simulink model "dspsdadc_fixpt"  (Simulink 8.3)
settings: Solver=ode5  SolverMode=SingleTasking  StartTime=0.0  StopTime=inf  MaxStep=1/512000  RelTol=1e-3  AbsTol=1e-6
libraries: dsparch4 x1, dspmlti4 x1, dspmisc x1
settings Model: Creator=The MathWorks Inc.  ExtModeTrigMode=oneshot  ExtModeArmWhenConnect=off  ExtModeAutoUpdateStatusClock=off
settings DataIOCC: LimitDataPoints=off  SignalLoggingSaveFormat=Dataset  SaveOutput=off  SaveTime=off  SignalLoggingName=logsOut
settings OptimizationCC: BlockReduction=off  BooleanDataType=off  ExpressionDepthLimit=2147483647  RollThreshold=2  InitFltsAndDblsToZero=on  EfficientMapNaN2IntZero=off
settings DebuggingCC: SaveWithParameterizedLinksMsg=none  SignalResolutionControl=TryResolveAllWithWarning  SolverPrmCheckMsg=none  MultiTaskDSMMsg=warning  MultiTaskCondExecSysMsg=none  IntegerOverflowMsg=none  ParameterPrecisionLossMsg=none  FcnCallInpInsideContextMsg=UseLocalSettings  StrictBusMsg=None  LoggingUnavailableSignals=none
settings HardwareCC: TargetUnknown=on
settings RTWCC: IncludeERTFirstTime=on
settings GRTTargetCC: TargetFcnLib=ansi_tfl_tmw.mat

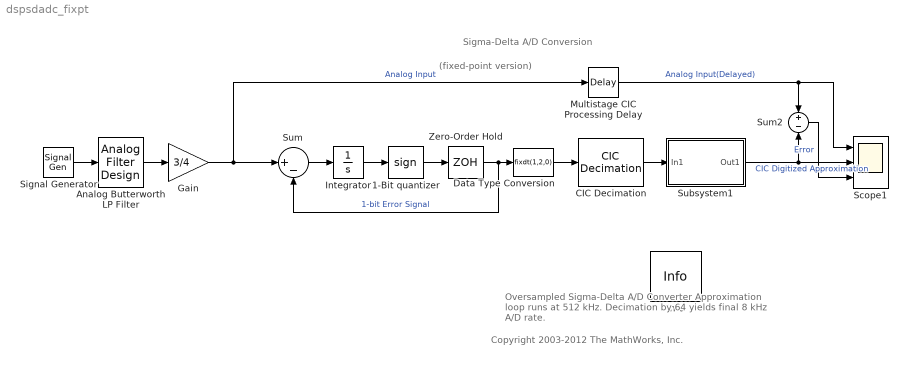
== system dspsdadc_fixpt ==
  note: Oversampled Sigma-Delta A/D Converter
      | Approximation loop runs at 512 kHz.
      | Decimation by 64 yields final 8 kHz A/D rate.
  note: Sigma-Delta A/D Conversion
  note: (fixed-point version)
  note: Copyright 2003-2012 The MathWorks, Inc.
  1-Bit quantizer : Signum
  Analog Butterworth LP Filter : dsparch4/Analog Filter Design  method=Butterworth  filttype=Lowpass  N=5  Wlo=2*pi*400  Whi=80  Rp=2  Rs=40
  CIC Decimation : dspmlti4/CIC Decimation  filtFrom=Dialog  filtobj=Hm_decim  ftype=Decimator  R=64  M=1  N=5  filterInternals=Full precision  BPS=[32 30 24 20 16 16 16 16 16 16]  FLPS=0  outputWordLength=16  outputFracLength=0  launchFVT=off  framing=Maintain input frame rate  RateOptions=Allow multirate processing
  Data Type Conversion : DataTypeConversion  OutDataTypeStr=fixdt(1,2,0)
  Gain : Gain  Gain=3/4  SaturateOnIntegerOverflow=on  OutDataTypeStr=Inherit: Same as input  ParamDataTypeStr=Inherit: Same as input
  Info : dspmisc/Info  SystemSampleTime=-1
  Integrator : Integrator
  Multistage CIC Processing Delay : TransportDelay  DelayTime=158/512000
  Scope1 : Scope  NumInputPorts=3
      settings: TimeRange=0.025  YMin=-1.1~-1.1~-0.25  YMax=1.1~1.1~0.25  MaxDataPoints=15000
  Signal Generator : SignalGenerator  WaveForm=square  Frequency=80
  Subsystem1 : Subsystem
      mask Display: disp('Rescaling for\nComparison')
  Sum : Sum  Inputs=|+-  SaturateOnIntegerOverflow=on  InputSameDT=on  OutDataTypeStr=Inherit: Same as first input
  Sum2 : Sum  Inputs=+-  RndMeth=Nearest  SaturateOnIntegerOverflow=on
  Zero-Order Hold : ZeroOrderHold  SampleTime=1/512000
  wires:
  Zero-Order Hold/1 -> Data Type Conversion/1, Sum/2  "1-bit Error Signal"
  1-Bit quantizer/1 -> Zero-Order Hold/1
  Sum/1 -> Integrator/1
  Integrator/1 -> 1-Bit quantizer/1
  Gain/1 -> Multistage CIC Processing Delay/1, Sum/1  "Analog Input"
  Analog Butterworth LP Filter/1 -> Gain/1
  Signal Generator/1 -> Analog Butterworth LP Filter/1
  Data Type Conversion/1 -> CIC Decimation/1
  CIC Decimation/1 -> Subsystem1/1(In1)
  Sum2/1 -> Scope1/3  "Error"
  Multistage CIC Processing Delay/1 -> Sum2/1, Scope1/1  "Analog Input(Delayed)"
  Subsystem1/1(Out1) -> Sum2/2, Scope1/2  "CIC Digitized Approximation"

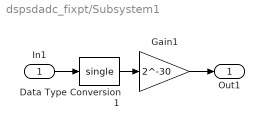
== system dspsdadc_fixpt/Subsystem1 ==
  In1 : Inport
  Data Type Conversion1 : DataTypeConversion  OutDataTypeStr=single
  Gain1 : Gain  Gain=2^-30  SaturateOnIntegerOverflow=on  OutDataTypeStr=Inherit: Same as input  ParamDataTypeStr=Inherit: Same as input
  Out1 : Outport
  wires:
  Data Type Conversion1/1 -> Gain1/1
  In1/1 -> Data Type Conversion1/1
  Gain1/1 -> Out1/1
